simulink model "Drone_simulation"  (R2024b)
settings: Solver=VariableStepAuto  StartTime=0.0  StopTime=t_stop  RelTol=1e-3
model workspace: external: MATLAB File Drone_parameters.m (data not in the file)
values from neighbouring files (symbols this model uses):
  d = 0.20    (= 0.2)    [Drone_parameters.m]
  disturbances_enabled = 0    [Drone_parameters.m]
  flight_mode = 3    [Drone_parameters.m]
  Fx_gust = 1.0    (= 1)    [Drone_parameters.m]
  Fy_gust = 1.0    (= 1)    [Drone_parameters.m]
  Fz_gust = 0.5    [Drone_parameters.m]
  inv_m = 0.3846    [Drone_parameters.m]
  Ixx = 0.05    [Drone_parameters.m]
  Iyy = 0.05    [Drone_parameters.m]
  Izz = 0.10    (= 0.1)    [Drone_parameters.m]
  Kd_phi = 0.5    [Drone_parameters.m]
  Kd_psi = 0.5    [Drone_parameters.m]
  Kd_theta = 0.28    [Drone_parameters.m]
  Kd_x = 0.16    [Drone_parameters.m]
  Kd_y = 0.16    [Drone_parameters.m]
  Kd_z = 4.5    [Drone_parameters.m]
  kf = 4.0e-5    (= 4e-05)    [Drone_parameters.m]
  Ki_phi = 0    [Drone_parameters.m]
  Ki_psi = 0    [Drone_parameters.m]
  Ki_theta = 0.28    [Drone_parameters.m]
  Ki_x = 0    [Drone_parameters.m]
  Ki_y = 0    [Drone_parameters.m]
  Ki_z = 0    [Drone_parameters.m]
  km = 1.0e-6    (= 1e-06)    [Drone_parameters.m]
  Kp_phi = 1.0    (= 1)    [Drone_parameters.m]
  Kp_psi = 1.0    (= 1)    [Drone_parameters.m]
  Kp_theta = 0.8    [Drone_parameters.m]
  Kp_x = 0.1    [Drone_parameters.m]
  Kp_y = 0.1    [Drone_parameters.m]
  Kp_z = 1.0    (= 1)    [Drone_parameters.m]
  mg = 25.5    [Drone_parameters.m]
  N_phi = 100    [Drone_parameters.m]
  N_psi = 100    [Drone_parameters.m]
  N_theta = 100    [Drone_parameters.m]
  N_x = 100    [Drone_parameters.m]
  N_y = 100    [Drone_parameters.m]
  N_z = 100    [Drone_parameters.m]
  omega_init = 399    [Drone_parameters.m]
  phi0 = 0    [Drone_parameters.m]
  phi_dot0 = 0    [Drone_parameters.m]
  phi_manual = 0    [Drone_parameters.m]
  pitch_pair_allocation = 1/(2*d)    (= 2.5)    [Drone_parameters.m]
  psi0 = 0    [Drone_parameters.m]
  psi_des = deg2rad(0)    [Drone_parameters.m]
  psi_dot0 = 0    [Drone_parameters.m]
  psi_hold = 0    [Drone_parameters.m]
  psi_manual = 0    [Drone_parameters.m]
  rad_to_deg = 180/pi    (= 57.2957795131)    [Drone_parameters.m]
  replay_collective_to_pair_thrust_N = 51.0    (= 51)    [Drone_parameters.m]
  replay_enabled = 0    [Drone_parameters.m]
  roll_motor_allocation = 1/(4*d)    (= 1.25)    [Drone_parameters.m]
  seed_phi = 104    [Drone_parameters.m]
  seed_psi = 106    [Drone_parameters.m]
  seed_theta = 105    [Drone_parameters.m]
  seed_x = 101    [Drone_parameters.m]
  seed_y = 102    [Drone_parameters.m]
  seed_z = 103    [Drone_parameters.m]
  sensor_noise_enabled = 0    [Drone_parameters.m]
  sensor_noise_tau_attitude = 0.10    (= 0.1)    [Drone_parameters.m]
  sensor_noise_tau_position = 0.20    (= 0.2)    [Drone_parameters.m]
  sensor_sample_time = 0.02    [Drone_parameters.m]
  sigma_phi = deg2rad(0.02)    [Drone_parameters.m]
  sigma_psi = deg2rad(0.05)    [Drone_parameters.m]
  sigma_theta = deg2rad(0.02)    [Drone_parameters.m]
  sigma_x = 0.002    [Drone_parameters.m]
  sigma_y = 0.002    [Drone_parameters.m]
  sigma_z = 0.001    [Drone_parameters.m]
  t_Fx_end = 11    [Drone_parameters.m]
  t_Fx_start = 10    [Drone_parameters.m]
  t_Fy_end = 16    [Drone_parameters.m]
  t_Fy_start = 15    [Drone_parameters.m]
  t_Fz_end = 21    [Drone_parameters.m]
  t_Fz_start = 20    [Drone_parameters.m]
  t_pitch_end = 30.5    [Drone_parameters.m]
  t_pitch_start = 30    [Drone_parameters.m]
  t_roll_end = 25.5    [Drone_parameters.m]
  t_roll_start = 25    [Drone_parameters.m]
  t_step_xy = 1    [Drone_parameters.m]
  t_step_yaw = 1    [Drone_parameters.m]
  t_step_z = 0    [Drone_parameters.m]
  t_yaw_end = 35.5    [Drone_parameters.m]
  t_yaw_start = 35    [Drone_parameters.m]
  tau_m = 0.05    [Drone_parameters.m]
  tau_pitch_gust = 0.01    [Drone_parameters.m]
  tau_roll_gust = 0.01    [Drone_parameters.m]
  tau_yaw_gust = 0.002    [Drone_parameters.m]
  theta0 = 0    [Drone_parameters.m]
  theta_dot0 = 0    [Drone_parameters.m]
  theta_manual = 0    [Drone_parameters.m]
  tilt_max = 0.1745    [Drone_parameters.m]
  Tmax = 12.5    [Drone_parameters.m]
  Tmin = 0    [Drone_parameters.m]
  vx0 = 0    [Drone_parameters.m]
  vy0 = 0    [Drone_parameters.m]
  vz0 = 0    [Drone_parameters.m]
  x0 = 0    [Drone_parameters.m]
  x_des = 4    [Drone_parameters.m]
  x_hold = 0    [Drone_parameters.m]
  x_manual = 0    [Drone_parameters.m]
  y0 = 0    [Drone_parameters.m]
  y_des = 2    [Drone_parameters.m]
  y_hold = 0    [Drone_parameters.m]
  y_manual = 0    [Drone_parameters.m]
  yaw_motor_allocation = kf/(4*km)    (= 10)    [Drone_parameters.m]
  z0 = 0    [Drone_parameters.m]
  z_des = 1    [Drone_parameters.m]
  z_hold = 1    [Drone_parameters.m]
  z_manual = 1    [Drone_parameters.m]
libraries: slpidlib x6
(part 2 of 2)

== system Drone_simulation/X_Position_Controller ==
  x_des : Inport
  x : Inport  Port=2
  Pitch_Command_Limit : Saturate  UpperLimit=tilt_max  LowerLimit=-tilt_max
  X_Position_Error : Sum  Inputs=+-|
  X_Position_PID : slpidlib/PID Controller  Controller=PID  Form=Parallel  TimeDomain=Continuous-time  UseExternalTs=off  SampleTime=-1  IntegratorMethod=Forward Euler  FilterMethod=Forward Euler  ControllerParametersSource=internal  P=Kp_x  I=Ki_x  UseKiTs=off  D=Kd_x  UseExternalDerivativeSource=off  N=N_x  UseFilter=on  TunerSelectOption=Transfer Function Based (PID Tuner App)  InitialConditionSource=internal  InitialConditionForIntegrator=0  InitialConditionForFilter=0  DifferentiatorICPrevScaledInput=0  ExternalReset=none  TrackingMode=off  Kt=1  LimitOutput=off  SatLimitsSource=internal  UpperSaturationLimit=inf  LowerSaturationLimit=-inf  LinearizeAsGain=on  AntiWindupMode=none  Kb=1  LimitIntegrator=off  UpperIntegratorSaturationLimit=inf  LowerIntegratorSaturationLimit=-inf  POutMin=[]  POutMax=[]  IOutMin=[]  IOutMax=[]  DOutMin=[]  DOutMax=[]  NOutMin=[]  NOutMax=[]  SumOutMin=[]  SumOutMax=[]  SaturationOutMin=[]  SaturationOutMax=[]  PParamMin=[]  PParamMax=[]  IParamMin=[]  IParamMax=[]  DParamMin=[]  DParamMax=[]  NParamMin=[]  NParamMax=[]  KbParamMin=[]  KbParamMax=[]  KtParamMin=[]  KtParamMax=[]  KbOutMin=[]  KbOutMax=[]  KtOutMin=[]  KtOutMax=[]  IntegratorOutMin=[]  IntegratorOutMax=[]  FilterOutMin=[]  FilterOutMax=[]  SumI1OutMin=[]  SumI1OutMax=[]  SumI2OutMin=[]  SumI2OutMax=[]  SumI3OutMin=[]  SumI3OutMax=[]  SumI4OutMin=[]  SumI4OutMax=[]  SumDOutMin=[]  SumDOutMax=[]  DifferentiatorOutMin=[]  DifferentiatorOutMax=[]  FilterDiffOutCoefMin=[]  FilterDiffOutCoefMax=[]  ReciprocalOutMin=[]  ReciprocalOutMax=[]  SumDenOutMin=[]  SumDenOutMax=[]  SumNumOutMin=[]  SumNumOutMax=[]  DivideOutMin=[]  DivideOutMax=[]  UdiffTsProdOutMin=[]  UdiffTsProdOutMax=[]  NTsProdOutMin=[]  NTsProdOutMax=[]  UintegralTsProdOutMin=[]  UintegralTsProdOutMax=[]  UngainTsProdOutMin=[]  UngainTsProdOutMax=[]  ClampingZeroOutDataTypeStr=Inherit: Inherit via back propagation  ClampingZeroOutMin=[]  ClampingZeroOutMax=[]  FilterDenConstantOutDataTypeStr=Inherit: Inherit via back propagation  FilterDenConstantOutMin=[]  FilterDenConstantOutMax=[]  PCopyOutDataTypeStr=Inherit: Inherit via back propagation  PCopyOutMin=[]  PCopyOutMax=[]  NCopyOutDataTypeStr=Inherit: Inherit via back propagation  NCopyOutMin=[]  NCopyOutMax=[]  IntegratorContinuousStateAttributes=''  IntegratorStateMustResolveToSignalObject=off  IntegratorRTWStateStorageClass=Auto  FilterContinuousStateAttributes=''  FilterStateMustResolveToSignalObject=off  FilterRTWStateStorageClass=Auto  ParallelPVariant=InternalParameters  IdealPVariant=Disabled  IVariant=InternalParameters  DVariant=InternalParameters  IntegratorVariant=Continuous  SatVariant=Disabled  AWVariant=Passthrough  PCopyVariant=Disabled  TRVariant=Disabled  FdbkBlocksVariant=Forward  IdealPFdbkVariant=Disabled  SatFdbkVariant=Disabled  DerivativeFilterVariant=ContFilter  NVariant=InternalParameters  NCopyVariant=Disabled  FilterICVariant=InternalICsFilter  IntegratorICVariant=InternalICs  ExternalResetVariant=Disabled  TRSumVariant=Passthrough  SumFdbkVariant=Disabled  SumVariant=Sum_PID  TsampFilterVariant=InternalTs  TsampNgainVariant=Passthrough  TsampIntegralVariant=Disabled_SignalSpec  ExternalSaturationOutDataTypeStr=Inherit: Same as second input  DerivativeSourceVariant=ErrorSignal  PreIntVariant=InternalPreInt
  theta_des : Outport
  wires:
  x_des/1 -> X_Position_Error/1
  X_Position_PID/1 -> Pitch_Command_Limit/1
  x/1 -> X_Position_Error/2
  X_Position_Error/1 -> X_Position_PID/1
  Pitch_Command_Limit/1 -> theta_des/1

== system Drone_simulation/Y_Position_Controller ==
  y : Inport
  y_des : Inport  Port=2
  Roll_Command_Limit : Saturate  UpperLimit=tilt_max  LowerLimit=-tilt_max
  Roll_Command_Sign : Gain  Gain=-1
  Y_Position_Error : Sum  Inputs=|-+
  Y_Position_PID : slpidlib/PID Controller  Controller=PID  Form=Parallel  TimeDomain=Continuous-time  UseExternalTs=off  SampleTime=-1  IntegratorMethod=Forward Euler  FilterMethod=Forward Euler  ControllerParametersSource=internal  P=Kp_y  I=Ki_y  UseKiTs=off  D=Kd_y  UseExternalDerivativeSource=off  N=N_y  UseFilter=on  TunerSelectOption=Transfer Function Based (PID Tuner App)  InitialConditionSource=internal  InitialConditionForIntegrator=0  InitialConditionForFilter=0  DifferentiatorICPrevScaledInput=0  ExternalReset=none  TrackingMode=off  Kt=1  LimitOutput=off  SatLimitsSource=internal  UpperSaturationLimit=inf  LowerSaturationLimit=-inf  LinearizeAsGain=on  AntiWindupMode=none  Kb=1  LimitIntegrator=off  UpperIntegratorSaturationLimit=inf  LowerIntegratorSaturationLimit=-inf  POutMin=[]  POutMax=[]  IOutMin=[]  IOutMax=[]  DOutMin=[]  DOutMax=[]  NOutMin=[]  NOutMax=[]  SumOutMin=[]  SumOutMax=[]  SaturationOutMin=[]  SaturationOutMax=[]  PParamMin=[]  PParamMax=[]  IParamMin=[]  IParamMax=[]  DParamMin=[]  DParamMax=[]  NParamMin=[]  NParamMax=[]  KbParamMin=[]  KbParamMax=[]  KtParamMin=[]  KtParamMax=[]  KbOutMin=[]  KbOutMax=[]  KtOutMin=[]  KtOutMax=[]  IntegratorOutMin=[]  IntegratorOutMax=[]  FilterOutMin=[]  FilterOutMax=[]  SumI1OutMin=[]  SumI1OutMax=[]  SumI2OutMin=[]  SumI2OutMax=[]  SumI3OutMin=[]  SumI3OutMax=[]  SumI4OutMin=[]  SumI4OutMax=[]  SumDOutMin=[]  SumDOutMax=[]  DifferentiatorOutMin=[]  DifferentiatorOutMax=[]  FilterDiffOutCoefMin=[]  FilterDiffOutCoefMax=[]  ReciprocalOutMin=[]  ReciprocalOutMax=[]  SumDenOutMin=[]  SumDenOutMax=[]  SumNumOutMin=[]  SumNumOutMax=[]  DivideOutMin=[]  DivideOutMax=[]  UdiffTsProdOutMin=[]  UdiffTsProdOutMax=[]  NTsProdOutMin=[]  NTsProdOutMax=[]  UintegralTsProdOutMin=[]  UintegralTsProdOutMax=[]  UngainTsProdOutMin=[]  UngainTsProdOutMax=[]  ClampingZeroOutDataTypeStr=Inherit: Inherit via back propagation  ClampingZeroOutMin=[]  ClampingZeroOutMax=[]  FilterDenConstantOutDataTypeStr=Inherit: Inherit via back propagation  FilterDenConstantOutMin=[]  FilterDenConstantOutMax=[]  PCopyOutDataTypeStr=Inherit: Inherit via back propagation  PCopyOutMin=[]  PCopyOutMax=[]  NCopyOutDataTypeStr=Inherit: Inherit via back propagation  NCopyOutMin=[]  NCopyOutMax=[]  IntegratorContinuousStateAttributes=''  IntegratorStateMustResolveToSignalObject=off  IntegratorRTWStateStorageClass=Auto  FilterContinuousStateAttributes=''  FilterStateMustResolveToSignalObject=off  FilterRTWStateStorageClass=Auto  ParallelPVariant=InternalParameters  IdealPVariant=Disabled  IVariant=InternalParameters  DVariant=InternalParameters  IntegratorVariant=Continuous  SatVariant=Disabled  AWVariant=Passthrough  PCopyVariant=Disabled  TRVariant=Disabled  FdbkBlocksVariant=Forward  IdealPFdbkVariant=Disabled  SatFdbkVariant=Disabled  DerivativeFilterVariant=ContFilter  NVariant=InternalParameters  NCopyVariant=Disabled  FilterICVariant=InternalICsFilter  IntegratorICVariant=InternalICs  ExternalResetVariant=Disabled  TRSumVariant=Passthrough  SumFdbkVariant=Disabled  SumVariant=Sum_PID  TsampFilterVariant=InternalTs  TsampNgainVariant=Passthrough  TsampIntegralVariant=Disabled_SignalSpec  ExternalSaturationOutDataTypeStr=Inherit: Same as second input  DerivativeSourceVariant=ErrorSignal  PreIntVariant=InternalPreInt
  phi_des : Outport
  wires:
  y/1 -> Y_Position_Error/1
  Y_Position_Error/1 -> Y_Position_PID/1
  y_des/1 -> Y_Position_Error/2
  Roll_Command_Sign/1 -> Roll_Command_Limit/1
  Y_Position_PID/1 -> Roll_Command_Sign/1
  Roll_Command_Limit/1 -> phi_des/1

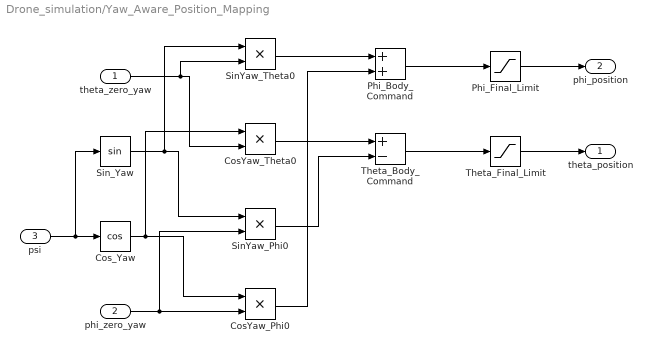
== system Drone_simulation/Yaw_Aware_Position_Mapping ==
  theta_zero_yaw : Inport
  phi_zero_yaw : Inport  Port=2
  psi : Inport  Port=3
  CosYaw_Phi0 : Product  Inputs=**
  CosYaw_Theta0 : Product  Inputs=**
  Cos_Yaw : Trigonometry  Operator=cos
  Phi_Body_Command : Sum
  Phi_Final_Limit : Saturate  UpperLimit=tilt_max  LowerLimit=-tilt_max
  SinYaw_Phi0 : Product  Inputs=**
  SinYaw_Theta0 : Product  Inputs=**
  Sin_Yaw : Trigonometry
  Theta_Body_Command : Sum  Inputs=+-
  Theta_Final_Limit : Saturate  UpperLimit=tilt_max  LowerLimit=-tilt_max
  theta_position : Outport
  phi_position : Outport  Port=2
  wires:
  Phi_Final_Limit/1 -> phi_position/1
  Phi_Body_Command/1 -> Phi_Final_Limit/1
  CosYaw_Phi0/1 -> Phi_Body_Command/2
  SinYaw_Theta0/1 -> Phi_Body_Command/1
  Theta_Final_Limit/1 -> theta_position/1
  Theta_Body_Command/1 -> Theta_Final_Limit/1
  SinYaw_Phi0/1 -> Theta_Body_Command/2
  CosYaw_Theta0/1 -> Theta_Body_Command/1
  phi_zero_yaw/1 -> SinYaw_Phi0/2, CosYaw_Phi0/2
  Sin_Yaw/1 -> SinYaw_Phi0/1, SinYaw_Theta0/1
  theta_zero_yaw/1 -> CosYaw_Theta0/2, SinYaw_Theta0/2
  Cos_Yaw/1 -> CosYaw_Theta0/1, CosYaw_Phi0/1
  psi/1 -> Cos_Yaw/1, Sin_Yaw/1

== system Drone_simulation/Yaw_Controller ==
  psi_des : Inport
  psi : Inport  Port=2
  Yaw_Error : Sum  Inputs=-+|
  Yaw_Motor_Allocation : Gain  Gain=yaw_motor_allocation
  Yaw_PID : slpidlib/PID Controller  Controller=PID  Form=Parallel  TimeDomain=Continuous-time  UseExternalTs=off  SampleTime=-1  IntegratorMethod=Forward Euler  FilterMethod=Forward Euler  ControllerParametersSource=internal  P=Kp_psi  I=Ki_psi  UseKiTs=off  D=Kd_psi  UseExternalDerivativeSource=off  N=N_psi  UseFilter=on  TunerSelectOption=Transfer Function Based (PID Tuner App)  InitialConditionSource=internal  InitialConditionForIntegrator=0  InitialConditionForFilter=0  DifferentiatorICPrevScaledInput=0  ExternalReset=none  TrackingMode=off  Kt=1  LimitOutput=off  SatLimitsSource=internal  UpperSaturationLimit=inf  LowerSaturationLimit=-inf  LinearizeAsGain=on  AntiWindupMode=none  Kb=1  LimitIntegrator=off  UpperIntegratorSaturationLimit=inf  LowerIntegratorSaturationLimit=-inf  POutMin=[]  POutMax=[]  IOutMin=[]  IOutMax=[]  DOutMin=[]  DOutMax=[]  NOutMin=[]  NOutMax=[]  SumOutMin=[]  SumOutMax=[]  SaturationOutMin=[]  SaturationOutMax=[]  PParamMin=[]  PParamMax=[]  IParamMin=[]  IParamMax=[]  DParamMin=[]  DParamMax=[]  NParamMin=[]  NParamMax=[]  KbParamMin=[]  KbParamMax=[]  KtParamMin=[]  KtParamMax=[]  KbOutMin=[]  KbOutMax=[]  KtOutMin=[]  KtOutMax=[]  IntegratorOutMin=[]  IntegratorOutMax=[]  FilterOutMin=[]  FilterOutMax=[]  SumI1OutMin=[]  SumI1OutMax=[]  SumI2OutMin=[]  SumI2OutMax=[]  SumI3OutMin=[]  SumI3OutMax=[]  SumI4OutMin=[]  SumI4OutMax=[]  SumDOutMin=[]  SumDOutMax=[]  DifferentiatorOutMin=[]  DifferentiatorOutMax=[]  FilterDiffOutCoefMin=[]  FilterDiffOutCoefMax=[]  ReciprocalOutMin=[]  ReciprocalOutMax=[]  SumDenOutMin=[]  SumDenOutMax=[]  SumNumOutMin=[]  SumNumOutMax=[]  DivideOutMin=[]  DivideOutMax=[]  UdiffTsProdOutMin=[]  UdiffTsProdOutMax=[]  NTsProdOutMin=[]  NTsProdOutMax=[]  UintegralTsProdOutMin=[]  UintegralTsProdOutMax=[]  UngainTsProdOutMin=[]  UngainTsProdOutMax=[]  ClampingZeroOutDataTypeStr=Inherit: Inherit via back propagation  ClampingZeroOutMin=[]  ClampingZeroOutMax=[]  FilterDenConstantOutDataTypeStr=Inherit: Inherit via back propagation  FilterDenConstantOutMin=[]  FilterDenConstantOutMax=[]  PCopyOutDataTypeStr=Inherit: Inherit via back propagation  PCopyOutMin=[]  PCopyOutMax=[]  NCopyOutDataTypeStr=Inherit: Inherit via back propagation  NCopyOutMin=[]  NCopyOutMax=[]  IntegratorContinuousStateAttributes=''  IntegratorStateMustResolveToSignalObject=off  IntegratorRTWStateStorageClass=Auto  FilterContinuousStateAttributes=''  FilterStateMustResolveToSignalObject=off  FilterRTWStateStorageClass=Auto  ParallelPVariant=InternalParameters  IdealPVariant=Disabled  IVariant=InternalParameters  DVariant=InternalParameters  IntegratorVariant=Continuous  SatVariant=Disabled  AWVariant=Passthrough  PCopyVariant=Disabled  TRVariant=Disabled  FdbkBlocksVariant=Forward  IdealPFdbkVariant=Disabled  SatFdbkVariant=Disabled  DerivativeFilterVariant=ContFilter  NVariant=InternalParameters  NCopyVariant=Disabled  FilterICVariant=InternalICsFilter  IntegratorICVariant=InternalICs  ExternalResetVariant=Disabled  TRSumVariant=Passthrough  SumFdbkVariant=Disabled  SumVariant=Sum_PID  TsampFilterVariant=InternalTs  TsampNgainVariant=Passthrough  TsampIntegralVariant=Disabled_SignalSpec  ExternalSaturationOutDataTypeStr=Inherit: Same as second input  DerivativeSourceVariant=ErrorSignal  PreIntVariant=InternalPreInt
  Yaw_cmd : Outport
  wires:
  Yaw_PID/1 -> Yaw_Motor_Allocation/1
  Yaw_Error/1 -> Yaw_PID/1
  psi/1 -> Yaw_Error/1
  psi_des/1 -> Yaw_Error/2
  Yaw_Motor_Allocation/1 -> Yaw_cmd/1

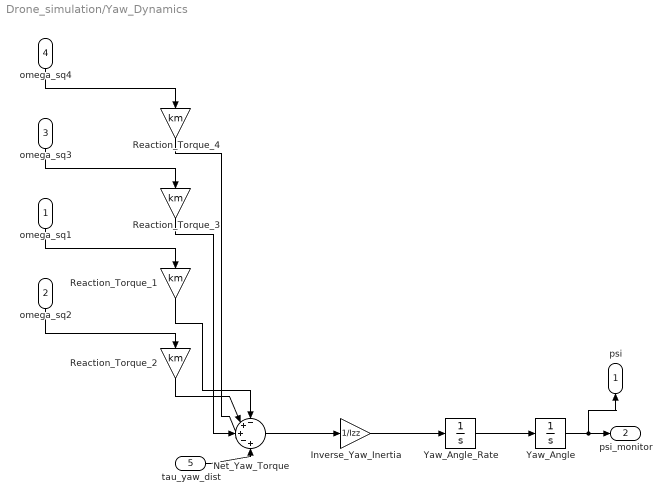
== system Drone_simulation/Yaw_Dynamics ==
  omega_sq1 : Inport
  omega_sq2 : Inport  Port=2
  omega_sq3 : Inport  Port=3
  omega_sq4 : Inport  Port=4
  tau_yaw_dist : Inport  Port=5
  Inverse_Yaw_Inertia : Gain  Gain=1/Izz
  Net_Yaw_Torque : Sum  Inputs=-++-+
  Reaction_Torque_{1..4} (4 alike) : Gain  Gain=km
  Yaw_Angle : Integrator  InitialCondition=psi0
  Yaw_Angle_Rate : Integrator  InitialCondition=psi_dot0
  psi : Outport
  psi_monitor : Outport  Port=2
  wires:
  Reaction_Torque_2/1 -> Net_Yaw_Torque/2
  omega_sq2/1 -> Reaction_Torque_2/1
  Reaction_Torque_4/1 -> Net_Yaw_Torque/4
  omega_sq1/1 -> Reaction_Torque_1/1
  omega_sq3/1 -> Reaction_Torque_3/1
  omega_sq4/1 -> Reaction_Torque_4/1
  Reaction_Torque_1/1 -> Net_Yaw_Torque/1
  Reaction_Torque_3/1 -> Net_Yaw_Torque/3
  Net_Yaw_Torque/1 -> Inverse_Yaw_Inertia/1
  Inverse_Yaw_Inertia/1 -> Yaw_Angle_Rate/1
  Yaw_Angle_Rate/1 -> Yaw_Angle/1
  Yaw_Angle/1 -> psi/1, psi_monitor/1
  tau_yaw_dist/1 -> Net_Yaw_Torque/5
